simulink model "doubts"  (R2020a)
settings: Solver=VariableStepAuto  StartTime=0.0  StopTime=10.0  RelTol=1e-3
settings Model: Creator=Kundan Patil  LastModifiedBy=Kundan Patil

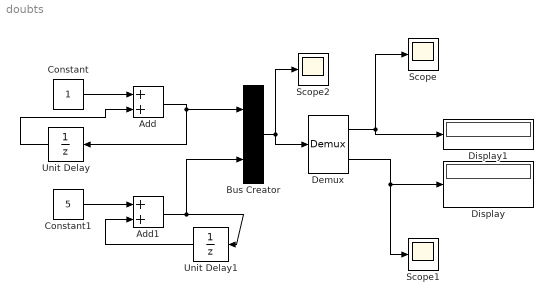
== system doubts ==
  Add : Sum
  Add1 : Sum
  Bus Creator : BusCreator  Inputs=2
  Constant : Constant
  Constant1 : Constant  Value=5
  Demux : Demux  Outputs=2
      settings: DisplayOption=none
  Display : Display
  Display1 : Display
  Scope : Scope
  Scope1 : Scope
  Scope2 : Scope
  Unit Delay : UnitDelay  SampleTime=-1  HasFrameUpgradeWarning=on
  Unit Delay1 : UnitDelay  SampleTime=-1  HasFrameUpgradeWarning=on
  wires:
  Constant/1 -> Add/1
  Constant1/1 -> Add1/1
  Add1/1 -> Bus Creator/2, Unit Delay1/1
  Unit Delay/1 -> Add/2
  Unit Delay1/1 -> Add1/2
  Add/1 -> Bus Creator/1, Unit Delay/1
  Bus Creator/1 -> Demux/1, Scope2/1
  Demux/2 -> Scope1/1, Display/1
  Demux/1 -> Scope/1, Display1/1
